simulink model "pmsm_initial_position"  (R2022b)
settings: Solver=FixedStepAuto  StartTime=0.0  StopTime=0.6  FixedStep=0.00002  MinStep=0.00025  RelTol=1e-3
values from neighbouring files (symbols this model uses):
  B = 0.0005    [pm_params.m]
  J = 0.0002    [pm_params.m]
  Lamda_f = 0.123    [pm_params.m]
  Ld = 0.0057    [pm_params.m]
  Lq = 0.0125    [pm_params.m]
  pole = 4    [pm_params.m]
  Rs = 1.2    [pm_params.m]
settings Model: Creator=jack  LastModifiedBy=jackyeh

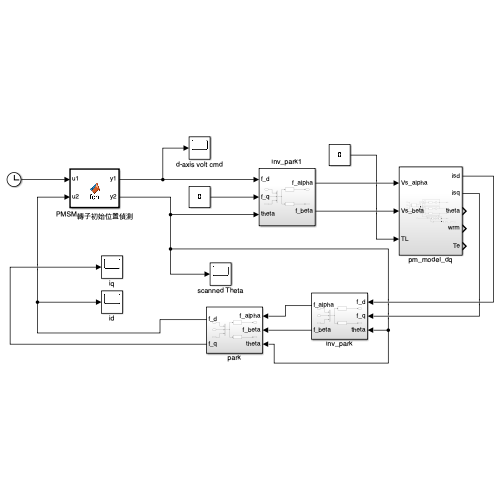
[thumbnail: Simulink's stored preview of the top-level diagram]
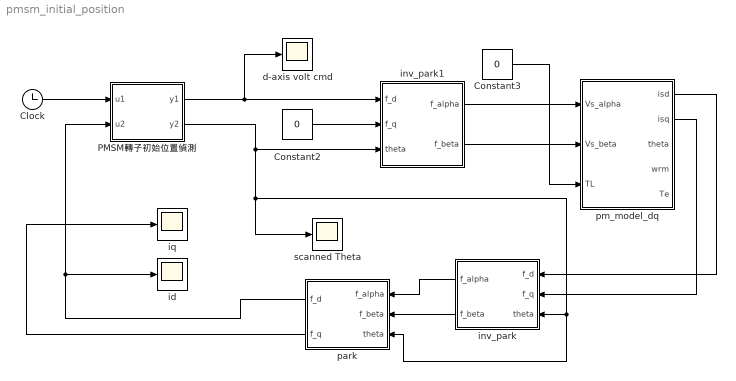
== system pmsm_initial_position ==
  Clock : Clock
  Constant2 : Constant  Value=0
  Constant3 : Constant  Value=0
  PMSM轉子初始位置偵測 : MATLAB Function  TreatAsAtomicUnit=on
  d-axis volt cmd : Scope
  id : Scope
  inv_park : Subsystem
  inv_park1 : Subsystem
  iq : Scope
  park : Subsystem
  pm_model_dq : Subsystem
  scanned Theta : Scope
  wires:
  pm_model_dq/2(isq) -> inv_park/2(f_q)
  pm_model_dq/1(isd) -> inv_park/1(f_d)
  Constant3/1 -> pm_model_dq/3(TL)
  PMSM轉子初始位置偵測/2(y2) -> inv_park/3(theta), park/3(theta), scanned Theta/1, inv_park1/3(theta)
  inv_park/1(f_alpha) -> park/1(f_alpha)
  inv_park/2(f_beta) -> park/2(f_beta)
  park/1(f_d) -> PMSM轉子初始位置偵測/2(u2), id/1
  park/2(f_q) -> iq/1
  inv_park1/1(f_alpha) -> pm_model_dq/1(Vs_alpha)
  inv_park1/2(f_beta) -> pm_model_dq/2(Vs_beta)
  Clock/1 -> PMSM轉子初始位置偵測/1(u1)
  PMSM轉子初始位置偵測/1(y1) -> d-axis volt cmd/1, inv_park1/1(f_d)
  Constant2/1 -> inv_park1/2(f_q)

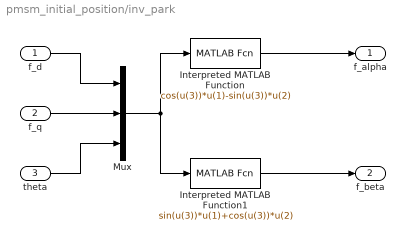
== system pmsm_initial_position/inv_park ==
  f_d : Inport
  f_q : Inport  Port=2
  theta : Inport  Port=3
  Interpreted MATLAB Function : MATLABFcn  MATLABFcn=cos(u(3))*u(1)-sin(u(3))*u(2)
  Interpreted MATLAB Function1 : MATLABFcn  MATLABFcn=sin(u(3))*u(1)+cos(u(3))*u(2)
  Mux : Mux  Inputs=3
  f_alpha : Outport
  f_beta : Outport  Port=2
  wires:
  Interpreted MATLAB Function/1 -> f_alpha/1
  f_d/1 -> Mux/1
  Mux/1 -> Interpreted MATLAB Function1/1, Interpreted MATLAB Function/1
  Interpreted MATLAB Function1/1 -> f_beta/1
  theta/1 -> Mux/3
  f_q/1 -> Mux/2

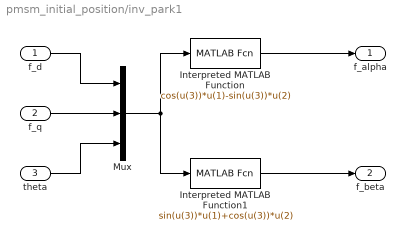
== system pmsm_initial_position/inv_park1 ==
  f_d : Inport
  f_q : Inport  Port=2
  theta : Inport  Port=3
  Interpreted MATLAB Function : MATLABFcn  MATLABFcn=cos(u(3))*u(1)-sin(u(3))*u(2)
  Interpreted MATLAB Function1 : MATLABFcn  MATLABFcn=sin(u(3))*u(1)+cos(u(3))*u(2)
  Mux : Mux  Inputs=3
  f_alpha : Outport
  f_beta : Outport  Port=2
  wires:
  f_q/1 -> Mux/2
  theta/1 -> Mux/3
  Interpreted MATLAB Function1/1 -> f_beta/1
  Mux/1 -> Interpreted MATLAB Function/1, Interpreted MATLAB Function1/1
  f_d/1 -> Mux/1
  Interpreted MATLAB Function/1 -> f_alpha/1

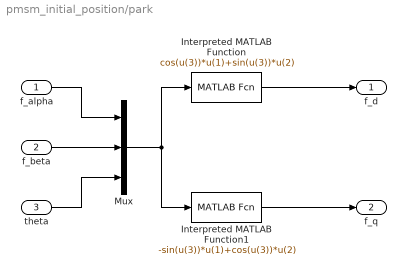
== system pmsm_initial_position/park ==
  f_alpha : Inport
  f_beta : Inport  Port=2
  theta : Inport  Port=3
  Interpreted MATLAB Function : MATLABFcn  MATLABFcn=cos(u(3))*u(1)+sin(u(3))*u(2)
  Interpreted MATLAB Function1 : MATLABFcn  MATLABFcn=-sin(u(3))*u(1)+cos(u(3))*u(2)
  Mux : Mux  Inputs=3
  f_d : Outport
  f_q : Outport  Port=2
  wires:
  Interpreted MATLAB Function/1 -> f_d/1
  f_alpha/1 -> Mux/1
  Mux/1 -> Interpreted MATLAB Function1/1, Interpreted MATLAB Function/1
  Interpreted MATLAB Function1/1 -> f_q/1
  theta/1 -> Mux/3
  f_beta/1 -> Mux/2

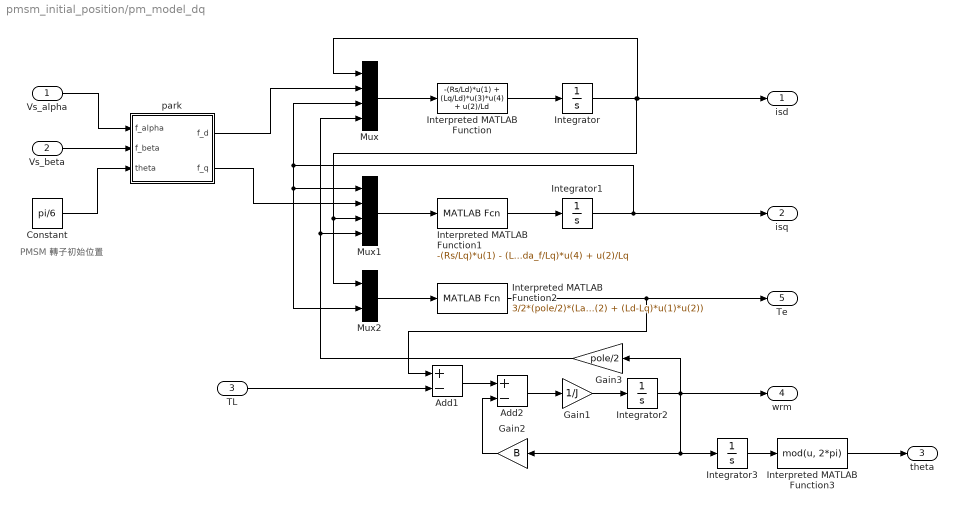
== system pmsm_initial_position/pm_model_dq ==
  note: PMSM 轉子初始位置
  Vs_alpha : Inport
  Vs_beta : Inport  Port=2
  TL : Inport  Port=3
  Add1 : Sum  Inputs=+-
  Add2 : Sum  Inputs=+-
  Constant : Constant  Value=pi/6
  Gain1 : Gain  Gain=1/J
  Gain2 : Gain  Gain=B
  Gain3 : Gain  Gain=pole/2
  Integrator{,1..3} (4 alike) : Integrator
  Interpreted MATLAB Function : MATLABFcn  MATLABFcn=-(Rs/Ld)*u(1) + (Lq/Ld)*u(3)*u(4) + u(2)/Ld
  Interpreted MATLAB Function1 : MATLABFcn  MATLABFcn=-(Rs/Lq)*u(1) - (Ld/Lq)*u(3)*u(4) - (Lamda_f/Lq)*u(4) + u(2)/Lq
  Interpreted MATLAB Function2 : MATLABFcn  MATLABFcn=3/2*(pole/2)*(Lamda_f*u(2) + (Ld-Lq)*u(1)*u(2))
  Interpreted MATLAB Function3 : MATLABFcn  MATLABFcn=mod(u, 2*pi)
  Mux : Mux
  Mux1 : Mux
  Mux2 : Mux  Inputs=2
  park : Subsystem
  isd : Outport
  isq : Outport  Port=2
  theta : Outport  Port=3
  wrm : Outport  Port=4
  Te : Outport  Port=5
  wires:
  Mux/1 -> Interpreted MATLAB Function/1
  Interpreted MATLAB Function1/1 -> Integrator1/1
  TL/1 -> Add1/2
  Integrator1/1 -> isq/1, Mux/3, Mux2/2, Mux1/1
  Interpreted MATLAB Function2/1 -> Te/1, Add1/1
  Gain3/1 -> Mux/4, Mux1/4
  Add2/1 -> Gain1/1
  Gain1/1 -> Integrator2/1
  Add1/1 -> Add2/1
  Mux2/1 -> Interpreted MATLAB Function2/1
  Interpreted MATLAB Function/1 -> Integrator/1
  Integrator/1 -> Mux2/1, Mux1/3, isd/1, Mux/1
  Integrator2/1 -> wrm/1, Gain3/1, Integrator3/1, Gain2/1
  Interpreted MATLAB Function3/1 -> theta/1
  Mux1/1 -> Interpreted MATLAB Function1/1
  Gain2/1 -> Add2/2
  Integrator3/1 -> Interpreted MATLAB Function3/1
  park/1(f_d) -> Mux/2
  park/2(f_q) -> Mux1/2
  Vs_alpha/1 -> park/1(f_alpha)
  Vs_beta/1 -> park/2(f_beta)
  Constant/1 -> park/3(theta)

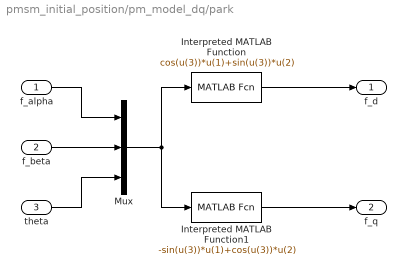
== system pmsm_initial_position/pm_model_dq/park ==
  f_alpha : Inport
  f_beta : Inport  Port=2
  theta : Inport  Port=3
  Interpreted MATLAB Function : MATLABFcn  MATLABFcn=cos(u(3))*u(1)+sin(u(3))*u(2)
  Interpreted MATLAB Function1 : MATLABFcn  MATLABFcn=-sin(u(3))*u(1)+cos(u(3))*u(2)
  Mux : Mux  Inputs=3
  f_d : Outport
  f_q : Outport  Port=2
  wires:
  Interpreted MATLAB Function/1 -> f_d/1
  f_alpha/1 -> Mux/1
  Mux/1 -> Interpreted MATLAB Function1/1, Interpreted MATLAB Function/1
  Interpreted MATLAB Function1/1 -> f_q/1
  theta/1 -> Mux/3
  f_beta/1 -> Mux/2

== matlab function pmsm_initial_position/PMSM轉子初始位置偵測 ==
  data: u1 input; y1 output; y2 output; u2 input
function [y1, y2] = fcn(u1, u2)
    Ts = 1e-4;
    theta_V=0:pi/12:2*pi;
    Um = 30;
    n=5; m=300;
    period = (n+m)*Ts;
    a = floor(u1/period); 
    b = mod(u1, period);
    if((u1 <= (a*period + n*Ts)) && (a<25))
      y1 = Um;
      y2 = theta_V(a+1);
    else
      y1 = 0;
      y2 = 0;
    end
